simulink model "Problem5_Sim"  (R2015b)
settings: Solver=ode45  StartTime=0.0  StopTime=Tmax  RelTol=1e-3
values from neighbouring files (symbols this model uses):
  A = [-1 1 0 0; 0 -1 0 0; 0 0 2 0; 0 0 0 -3]    [Problem5.m]
  B = [0 1; 1 0; 0 0; 1 0]    [Problem5.m]
  C = [0 1 0 1; 1 0 0 0]    [Problem5.m]
  D = [0 0;0 0]    [Problem5.m]
  x0 = [1 1 1 1]    [Problem5.m]
settings Model: Creator=Dana  LastModifiedBy=dmartin_a
settings DataIOCC: SaveFormat=Array
settings HardwareCC: ProdBitPerPointer=32  ProdLargestAtomicFloat=None  ProdIntDivRoundTo=Undefined  ProdEndianess=Unspecified  ProdWordSize=32  ProdHWDeviceType=32-bit Generic
settings GRTTargetCC: GeneratePreprocessorConditionals=Disable all
settings ConfigComp: CovModelRefEnable=Off

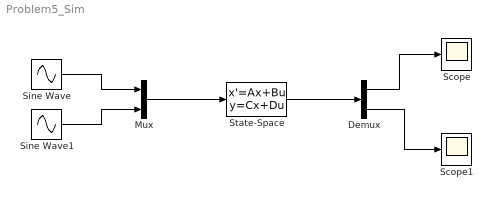
== system Problem5_Sim ==
  Demux : Demux  Outputs=2
  Mux : Mux  Inputs=2
  Scope : Scope
  Scope1 : Scope
  Sine Wave : Sin  SampleTime=0
  Sine Wave1 : Sin  SampleTime=0
  State-Space : StateSpace  A=A  B=B  C=C  D=D  X0=x0
  wires:
  State-Space/1 -> Demux/1
  Demux/1 -> Scope/1
  Demux/2 -> Scope1/1
  Mux/1 -> State-Space/1
  Sine Wave/1 -> Mux/1
  Sine Wave1/1 -> Mux/2
